simulink model "sltest_ratelim"  (R2026a)
settings: Solver=FixedStepDiscrete  StopTime=2  FixedStep=0.02  EnableMultiTasking=on
model workspace (MAT data in the model file):
  t_gain = [0; 2]
  t_neg = [0; 2]
  t_pos = [0; 1; 1; 2]
  u_gain = [0; 4]
  u_neg = [0; 0]
  u_pos = [0.02; 0.02; 0.1; 0.1]
settings Model: RequirementInfo=9  ExtModeAutoUpdateStatusClock=off  Creator=The MathWorks, Inc.  LastModifiedBy=The MathWorks, Inc.
settings OptimizationCC: InitFltsAndDblsToZero=on
settings DebuggingCC: SaveWithParameterizedLinksMsg=none  SignalResolutionControl=TryResolveAllWithWarning  MultiTaskDSMMsg=warning  MultiTaskCondExecSysMsg=none
settings HardwareCC: ProdHWDeviceType=32-bit Generic  TargetUnknown=on
settings GRTTargetCC: TargetFcnLib=ansi_tfl_tmw.mat  CombineOutputUpdateFcns=off  GRTInterface=on

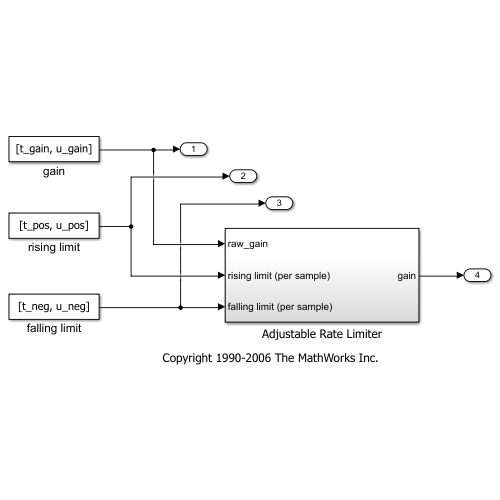
[thumbnail: Simulink's stored preview of the top-level diagram]
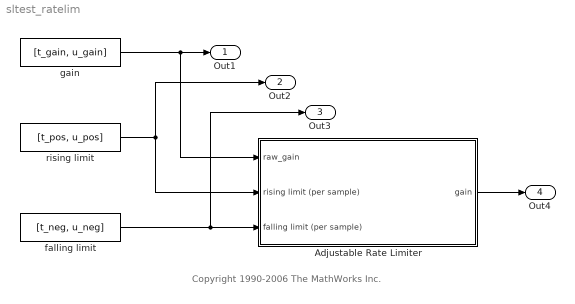
== system sltest_ratelim ==
  note: Copyright 1990-2006 The MathWorks Inc.
  Adjustable Rate Limiter : Subsystem
  falling limit : FromWorkspace  VariableName=[t_neg, u_neg]  ZeroCross=off
  gain : FromWorkspace  VariableName=[t_gain, u_gain]  ZeroCross=off
  rising limit : FromWorkspace  VariableName=[t_pos, u_pos]  ZeroCross=off
  Out1 : Outport
  Out2 : Outport  Port=2
  Out3 : Outport  Port=3
  Out4 : Outport  Port=4
  wires:
  falling limit/1 -> Adjustable Rate Limiter/3(falling limit (per sample)), Out3/1
  rising limit/1 -> Adjustable Rate Limiter/2(rising limit (per sample)), Out2/1
  gain/1 -> Out1/1, Adjustable Rate Limiter/1(raw_gain)
  Adjustable Rate Limiter/1(gain) -> Out4/1

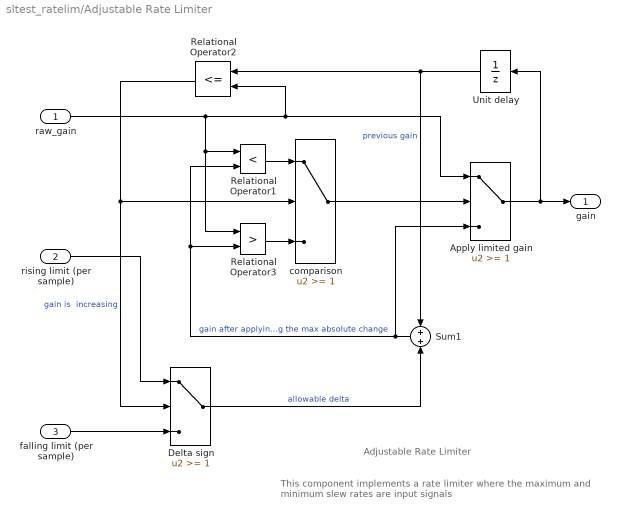
== system sltest_ratelim/Adjustable Rate Limiter ==
  note: This component implements a rate limiter where the
      | maximum and minimum slew rates are input signals
  note: Adjustable Rate Limiter
  raw_gain : Inport
  rising limit (per sample) : Inport  Port=2
  falling limit (per sample) : Inport  Port=3
  Apply limited gain : Switch  Threshold=1
  Delta sign : Switch  Threshold=1
  Relational Operator1 : RelationalOperator  Operator=<
  Relational Operator2 : RelationalOperator  Operator=<=
  Relational Operator3 : RelationalOperator  Operator=>
  Sum1 : Sum  InputSameDT=on  SaturateOnIntegerOverflow=on  OutDataTypeStr=Inherit: Same as first input
  Unit delay : UnitDelay  SampleTime=.02
  comparison : Switch  Threshold=1
  gain : Outport
  wires:
  Sum1/1 -> Apply limited gain/3, Relational Operator3/2, Relational Operator1/2  "gain after applying the max absolute change"
  comparison/1 -> Apply limited gain/2
  Relational Operator1/1 -> comparison/1
  Relational Operator3/1 -> comparison/3
  Delta sign/1 -> Sum1/2  "allowable delta"
  Relational Operator2/1 -> comparison/2, Delta sign/2  "gain is  increasing"
  falling limit (per sample)/1 -> Delta sign/3
  rising limit (per sample)/1 -> Delta sign/1
  Unit delay/1 -> Sum1/1, Relational Operator2/1  "previous gain"
  raw_gain/1 -> Relational Operator1/1, Relational Operator3/1, Relational Operator2/2, Apply limited gain/1
  Apply limited gain/1 -> Unit delay/1, gain/1
